simulink model "quad"  (Simulink 9.1)
settings: Solver=ode23  StartTime=0.0  StopTime=param.tf  MaxStep=0.1  RelTol=1e-4  EnableMultiTasking=on
undefined symbols (not defined in the file or in its folder): param
libraries: simulink_extras x4
settings Model: Creator=tristan  LastModifiedBy=Sam
settings DataIOCC: LimitDataPoints=on  SignalLoggingSaveFormat=ModelDataLogs
settings OptimizationCC: ExpressionDepthLimit=2147483647
settings DebuggingCC: SolverPrmCheckMsg=warning  FcnCallInpInsideContextMsg=warning  StateNameClashWarn=warning
settings GRTTargetCC: GeneratePreprocessorConditionals=Disable all

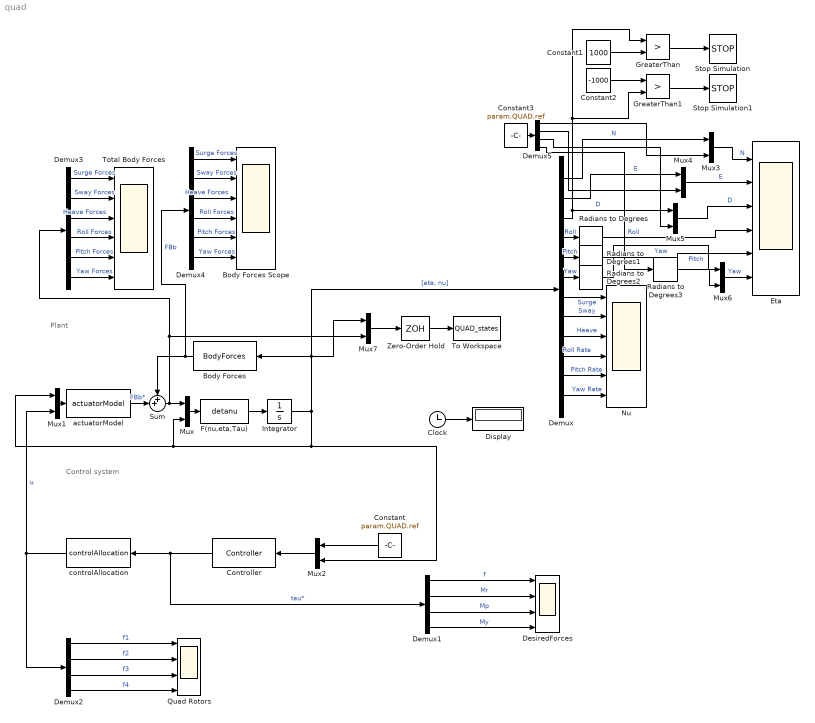
== system quad ==
  note: Control system
  note: Plant
  Body Forces : MATLABFcn  MATLABFcn=BodyForces  OutputDimensions=6
  "Body Forces Scope " : Scope  NumInputPorts=6
  Clock : Clock
  Constant : Constant  Value=param.QUAD.ref
  Constant1 : Constant  Value=1000
  Constant2 : Constant  Value=-1000
  Constant3 : Constant  Value=param.QUAD.ref
  Controller : MATLABFcn  MATLABFcn=Controller  OutputDimensions=4
  Demux : Demux  Outputs=12
  Demux1 : Demux
  Demux2 : Demux
  Demux3 : Demux  Outputs=6
  Demux4 : Demux  Outputs=6
  Demux5 : Demux
  DesiredForces : Scope  NumInputPorts=4
  Display : Display
  Eta : Scope  NumInputPorts=6
  F(nu,eta,Tau) : MATLABFcn  MATLABFcn=detanu  OutputDimensions=12
  GreaterThan : RelationalOperator  Operator=>  OutDataTypeStr=boolean  RndMeth=Simplest
  GreaterThan1 : RelationalOperator  Operator=>  OutDataTypeStr=boolean  RndMeth=Simplest
  Integrator : Integrator  InitialCondition=param.QUAD.X0
  Mux{,1..7} (8 alike) : Mux  Inputs=2
  Nu : Scope  NumInputPorts=6
  Quad Rotors : Scope  NumInputPorts=4
  Radians to Degrees{,1..3} (4 alike) : simulink_extras/Transformations/Radians to Degrees
  Stop Simulation : Stop
  Stop Simulation1 : Stop
  Sum : Sum  Inputs=++|
  To Workspace : ToWorkspace  VariableName=QUAD_states  SaveFormat=Timeseries  SampleTime=-1
  Total Body Forces : Scope  NumInputPorts=6
  Zero-Order Hold : ZeroOrderHold  SampleTime=1/param.sensor_sample_rate
  actuatorModel : MATLABFcn  MATLABFcn=actuatorModel  OutputDimensions=6
  controlAllocation : MATLABFcn  MATLABFcn=controlAllocation  OutputDimensions=4
  wires:
  Controller/1 -> controlAllocation/1, Demux1/1  "tau*"
  Demux1/1 -> DesiredForces/1  "f"
  Demux1/2 -> DesiredForces/2  "Mr"
  Mux/1 -> F(nu,eta,Tau)/1
  F(nu,eta,Tau)/1 -> Integrator/1
  Integrator/1 -> Mux7/1, Body Forces/1, Demux/1, Mux2/2, Mux1/1, Mux/2  "[eta; nu]"
  Demux1/3 -> DesiredForces/3  "Mp"
  actuatorModel/1 -> Sum/2  "FBb*"
  controlAllocation/1 -> Mux1/2, Demux2/1  "u"
  Demux1/4 -> DesiredForces/4  "My"
  Demux/1 -> Mux3/1  "N"
  Demux/2 -> Mux4/1  "E"
  Demux/3 -> Mux5/1, GreaterThan1/2, GreaterThan/1  "D"
  Demux/4 -> Radians to Degrees/1  "Roll"
  Demux/5 -> Radians to Degrees1/1  "Pitch"
  Demux/6 -> Radians to Degrees2/1  "Yaw"
  Demux/7 -> Nu/1  "Surge"
  Demux/8 -> Nu/2  "Sway"
  Demux/9 -> Nu/3  "Heave"
  Demux/10 -> Nu/4  "Roll Rate"
  Demux/11 -> Nu/5  "Pitch Rate"
  Demux/12 -> Nu/6  "Yaw Rate"
  Demux2/4 -> Quad Rotors/4  "f4"
  Demux2/3 -> Quad Rotors/3  "f3"
  Demux2/2 -> Quad Rotors/2  "f2"
  Demux2/1 -> Quad Rotors/1  "f1"
  Clock/1 -> Display/1
  Sum/1 -> Mux7/2, Demux3/1, Mux/1
  Body Forces/1 -> Demux4/1, Sum/1  "FBb"
  Demux3/1 -> Total Body Forces/1  "Surge Forces"
  Demux3/2 -> Total Body Forces/2  "Sway Forces"
  Demux3/3 -> Total Body Forces/3  "Heave Forces"
  Demux3/4 -> Total Body Forces/4  "Roll Forces"
  Demux3/5 -> Total Body Forces/5  "Pitch Forces"
  Demux3/6 -> Total Body Forces/6  "Yaw Forces"
  Mux1/1 -> actuatorModel/1
  Mux2/1 -> Controller/1
  Constant/1 -> Mux2/1
  Radians to Degrees1/1 -> Eta/5  "Pitch"
  Radians to Degrees2/1 -> Mux6/1  "Yaw"
  Demux4/6 -> "Body Forces Scope "/6  "Yaw Forces"
  Demux4/5 -> "Body Forces Scope "/5  "Pitch Forces"
  Demux4/4 -> "Body Forces Scope "/4  "Roll Forces"
  Demux4/3 -> "Body Forces Scope "/3  "Heave Forces"
  Demux4/2 -> "Body Forces Scope "/2  "Sway Forces"
  Demux4/1 -> "Body Forces Scope "/1  "Surge Forces"
  GreaterThan/1 -> Stop Simulation/1
  Constant1/1 -> GreaterThan/2
  Constant2/1 -> GreaterThan1/1
  GreaterThan1/1 -> Stop Simulation1/1
  Mux3/1 -> Eta/1  "N"
  Mux4/1 -> Eta/2  "E"
  Mux5/1 -> Eta/3  "D"
  Constant3/1 -> Demux5/1
  Demux5/1 -> Mux3/2
  Demux5/2 -> Mux4/2
  Demux5/3 -> Mux5/2
  Mux6/1 -> Eta/6  "Yaw"
  Demux5/4 -> Radians to Degrees3/1
  Radians to Degrees3/1 -> Mux6/2
  Radians to Degrees/1 -> Eta/4  "Roll"
  Mux7/1 -> Zero-Order Hold/1
  Zero-Order Hold/1 -> To Workspace/1
